simulink model "ERRK"  (R2025a)
settings: Solver=VariableStepAuto  StartTime=0.0  StopTime=10.0  MaxStep=1/50  RelTol=1e-3
settings Model: Creator=Szalay  LastModifiedBy=Szalay

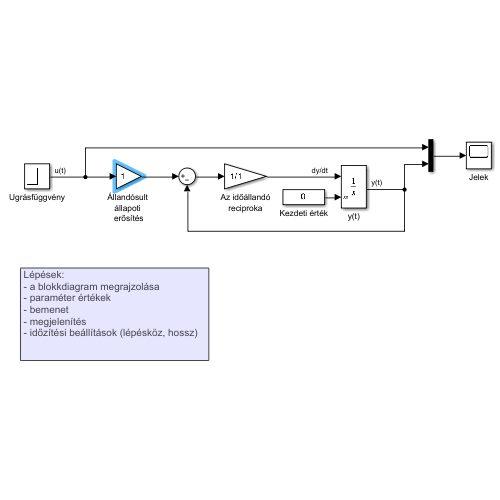
[thumbnail: Simulink's stored preview of the top-level diagram]
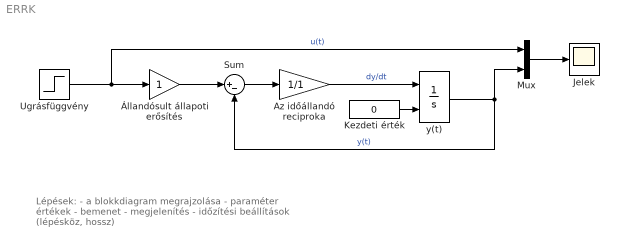
== system ERRK ==
  note: Lépések:
      | - a blokkdiagram megrajzolása
      | - paraméter értékek
      | - bemenet
      | - megjelenítés
      | - időzítési beállítások (lépésköz, hossz)
  Az időállandó reciproka : Gain  Gain=1/1
  Jelek : Scope
      settings: ActiveDisplayYMinimum=-0.12499999999999997  ActiveDisplayYMaximum=1.125
  Kezdeti érték : Constant  Value=0
  Mux : Mux  Inputs=2
  Sum : Sum  Inputs=|+-
  Ugrásfüggvény : Step  Time=0  SampleTime=0
  y(t) : Integrator  InitialConditionSource=external
  Állandósult állapoti erősítés : Gain
  wires:
  Az időállandó reciproka/1 -> y(t)/1  "dy/dt"
  Sum/1 -> Az időállandó reciproka/1
  y(t)/1 -> Mux/2, Sum/2  "y(t)"
  Kezdeti érték/1 -> y(t)/2
  Állandósult állapoti erősítés/1 -> Sum/1
  Ugrásfüggvény/1 -> Állandósult állapoti erősítés/1, Mux/1  "u(t)"
  Mux/1 -> Jelek/1
